simulink model "VSD_Model"  (R2022a)
settings: Solver=VariableStepAuto  StartTime=0.0  StopTime=60
values from neighbouring files (symbols this model uses):
  Bm = 7.33*10^-8/(2*pi)    (= 1.16660573286e-08)    [VSD_Motors_initialization.m]
  fit_Cp_tail = @(u)feval(f_Cp_tail,u)    [VSD_Propellerfitting_tail.m]
  fit_Ct_tail = @(u)feval(f_Ct_tail,u)    [VSD_Propellerfitting_tail.m]
  fit_Pe_tail = @(u)feval(f_Pe_tail,u)    [VSD_Propellerfitting_tail.m]
  fit_Tl_tail = @(u)feval(f_Tl_tail,u)    [VSD_Propellerfitting_tail.m]
  Jm = 1.72 *10^-6    (= 1.72e-06)    [VSD_Motors_initialization.m]
  Ke = Km    (= 0.00118)    [VSD_Motors_initialization.m]
  Km = 1.18*10^-3    (= 0.00118)    [VSD_Motors_initialization.m]
  La = 0.274*10^-3    (= 0.000274)    [VSD_Motors_initialization.m]
  Q = 1e-6    (= 1e-06)    [VSD_initialization.m]
  R = 0.486    [VSD_Motors_initialization.m]    (also in VSD_initialization.m = 0.001)
  Ts = 1e-4    (= 0.0001)    [VSD_initialization.m]    (also in myStateTransitionFcn.m = 0.01)
  x0 = [0;0;0;0;0;0;0;0;0;0;0;0]    [VSD_SystemCheck.m]    (also in VSD_initialization.m = [0,0,0,0,0,0,0,0,0,0,0,0])
undefined symbols (not defined in the file or in its folder): Continuous, Time
libraries: slpidlib x7, simulink x7, sharedTrackingLibrary x3, ctrlSharedLib x1
(part 1 of 2)
settings Model: Creator=luca9  LastModifiedBy=luca9
settings SolverCC: AlgebraicLoopSolver=TrustRegion
settings DebuggingCC: UnconnectedInputMsg=warning  UnconnectedOutputMsg=warning  UnconnectedLineMsg=warning
settings RTWCC: DLArmComputeVersion=19.05

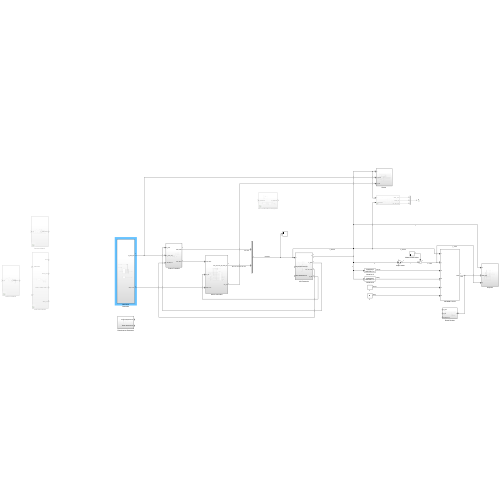
[thumbnail: Simulink's stored preview of the top-level diagram]
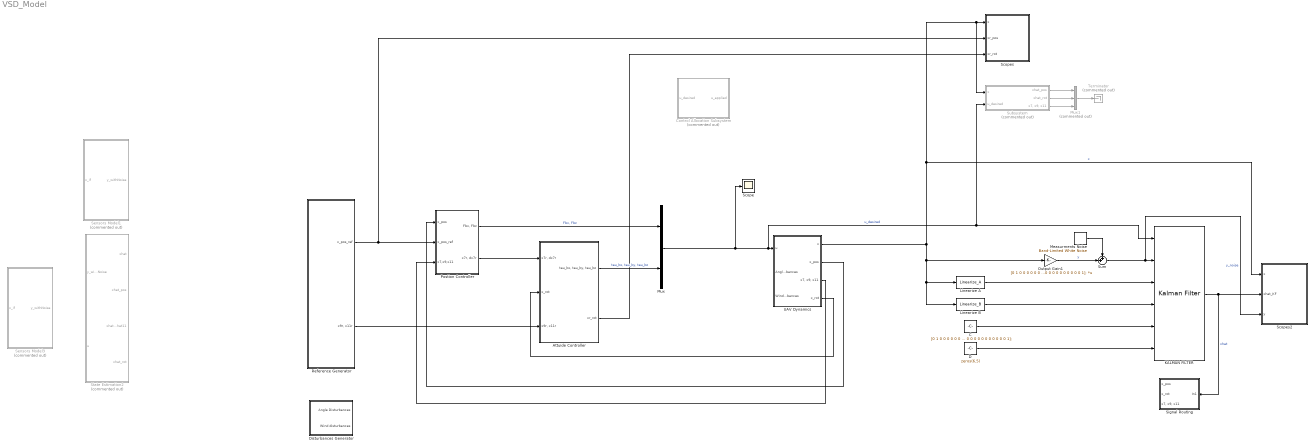
== system VSD_Model ==
  Attuide Controller : Subsystem
  C : Constant  Value=|  VectorParams1D=off
      | [0 1 0 0 0 0 0 0 0 0 0 0;
      |      0 0 0 1 0 0 0 0 0 0 0 0;
      |      0 0 0 0 0 1 0 0 0 0 0 0;
      |      0 0 0 0 0 0 0 1 0 0 0 0;
      |      0 0 0 0 0 0 0 0 0 1 0 0;
      |      0 0 0 0 0 0 0 0 0 0 0 1];
  Control Allocation Subsystem : Subsystem  Commented=on
  D : Constant  Value=zeros(6,5)  VectorParams1D=off
  Disturbances Generator : Subsystem
  KALMAN FILTER : ctrlSharedLib/Kalman Filter  TimeDomain=Continuous-Time  UseCurrentEstimator=on  ModelSource=Input port  ModelSourceVariable=ss(0.95,1,1,0,1)  A=0.95  B=1  C=1  D=0  NumberOfStates=12  NumberOfInputs=5  NumberOfOutputs=6  InitialEstimateSource=Dialog  X0=x0  P0=10^-2*eye(12)  UseK=off  UseGH=off  NumberOfProcessNoiseInputs=1  G=1  TimeInvariantG=on  H=0  TimeInvariantH=on  Q=Q*eye(12)  TimeInvariantQ=on  R=R*eye(6)  TimeInvariantR=on  N=0  TimeInvariantN=on  AddInputPort=on  AddEnablePort=off  OutputEstimatedY=off  OutputP=off  Ts=-1
  Linearize A : MATLABFcn  MATLABFcn=Linearize_A  OutputDimensions=[12,12]  Output1D=off
  Linearize B : MATLABFcn  MATLABFcn=Linearize_B  OutputDimensions=[12,5]  Output1D=off
  "Measurments Noise " : simulink/Sources/Band-Limited White Noise  Cov=R*Ts  Ts=Ts  seed=[23341]
  Mux : Mux  Inputs=2
  Mux1 : Mux  Commented=on  Inputs=3
  Output Gain1 : Gain  Gain=|  Multiplication=Matrix(K*u)
      | [0 1 0 0 0 0 0 0 0 0 0 0;
      |      0 0 0 1 0 0 0 0 0 0 0 0;
      |      0 0 0 0 0 1 0 0 0 0 0 0;
      |      0 0 0 0 0 0 0 1 0 0 0 0;
      |      0 0 0 0 0 0 0 0 0 1 0 0;
      |      0 0 0 0 0 0 0 0 0 0 0 1];
  Postion Controller : Subsystem
  Reference Generator : Subsystem
  Scope : Scope
  Scopes : Subsystem
  Scopes2 : Subsystem
  Sensors Model1 : Subsystem  Commented=on
  Sensors Model3 : Subsystem  Commented=on
  Signal Routing : Subsystem
  State Estimation2 : Subsystem  Commented=on
  Subsystem : Subsystem  Commented=on
  Sum : Sum  Inputs=++|
  Terminator : Terminator  Commented=on
  UAV Dynamics : Subsystem
  wires:
  Postion Controller/2("x7r, dx7r") -> Attuide Controller/1("x7r, dx7r")
  Mux/1 -> Scope/1, Subsystem/2(u_desired), KALMAN FILTER/1, UAV Dynamics/1(u)  "u_desired"
  Attuide Controller/1("tau_bx, tau_by, tau_bz") -> Mux/2  "tau_bx, tau_by, tau_bz"
  Postion Controller/1("Fbx, Fbz") -> Mux/1  "Fbx, Fbz"
  Reference Generator/1(x_pos_ref) -> Scopes/2(xr_pos), Postion Controller/2(x_pos_ref)
  Reference Generator/2("x9r, x11r") -> Attuide Controller/3("x9r, x11r")
  UAV Dynamics/1(x) -> Subsystem/1(x), Scopes/1(x), Scopes2/1(x), Output Gain1/1, Linearize B/1, Linearize A/1  "x"
  Attuide Controller/2(xr_rot) -> Scopes/3(xr_rot)
  Linearize A/1 -> KALMAN FILTER/3
  Linearize B/1 -> KALMAN FILTER/4
  D/1 -> KALMAN FILTER/6
  KALMAN FILTER/1 -> Scopes2/2(xhat_KF), Signal Routing/1(In1)  "xhat"
  Output Gain1/1 -> Sum/2  "y"
  Sum/1 -> Scopes2/3(y), KALMAN FILTER/2  "y_noise"
  "Measurments Noise "/1 -> Sum/1
  Subsystem/2(xhat_rot) -> Mux1/2
  Subsystem/1(xhat_pos) -> Mux1/1
  Subsystem/3("x7, x9, x11") -> Mux1/3
  Mux1/1 -> Terminator/1
  C/1 -> KALMAN FILTER/5
  UAV Dynamics/2(x_pos) -> Postion Controller/1(x_pos)
  UAV Dynamics/4(x_rot) -> Attuide Controller/2(x_rot)
  UAV Dynamics/3("x7, x9, x11") -> Postion Controller/3(" x7,x9,x11")

== system VSD_Model/Attuide Controller ==
  "x7r, dx7r" : Inport
  x_rot : Inport  Port=2
  "x9r, x11r" : Inport  Port=3
  Attitude Controller : MATLAB Function  TreatAsAtomicUnit=on
  Constant : Constant  Value=0
  Constant1 : Constant  Value=0
  Demux : Demux  Outputs=2
  Demux1 : Demux  Outputs=2
  Mux : Mux  Inputs=3
  Mux1 : Mux  Inputs=6
  Scope : Scope
  To Workspace : ToWorkspace  VariableName=s  SampleTime=-1
  "tau_bx, tau_by, tau_bz" : Outport
  xr_rot : Outport  Port=2
  wires:
  x_rot/1 -> Attitude Controller/1(x_rot)
  "x7r, dx7r"/1 -> Demux/1
  Demux/1 -> Attitude Controller/2(x7r), Mux1/1  "x7r"
  Demux/2 -> Attitude Controller/3(dx7r), Mux1/2  "dx7r"
  Demux1/1 -> Attitude Controller/4(x9r), Mux1/3  "x9r"
  "x9r, x11r"/1 -> Demux1/1
  Demux1/2 -> Mux1/5, Attitude Controller/6(x11r)
  Constant/1 -> Attitude Controller/5(dx9r), Mux1/4  "dx9r"
  Constant1/1 -> Attitude Controller/7(dx11r), Mux1/6
  Mux/1 -> "tau_bx, tau_by, tau_bz"/1
  Attitude Controller/2(u5) -> Mux/2
  Attitude Controller/1(u4) -> Mux/1
  Attitude Controller/3(u6) -> Mux/3
  Mux1/1 -> xr_rot/1
  Attitude Controller/4(s) -> To Workspace/1, Scope/1

== system VSD_Model/Control Allocation Subsystem ==
  u_desired : Inport
  Control allocation : Subsystem  Commented=on
  DC Motors : Subsystem  Commented=on
  Mux3 : Mux  Commented=on  Inputs=2
  Mux4 : Mux  Commented=on
  Scope1 : Scope  Commented=on  NumInputPorts=2
  Step{1..6} (6 alike) : Step  Commented=on  Time=0  After=0  SampleTime=0
  u_applied : Outport
  wires:
  DC Motors/1(y) -> Scope1/2, u_applied/1  "u_applied"
  Control allocation/7(alpha_r) -> DC Motors/7(alpha_r)
  Control allocation/2(W2) -> DC Motors/2(W2)
  Control allocation/6(alpha_l) -> DC Motors/6(alpha_l)
  Step4/1 -> Mux4/2
  Step6/1 -> Mux4/4
  u_desired/1 -> Control allocation/1(u), Scope1/1
  Control allocation/4(W4) -> DC Motors/4(W4)
  Control allocation/5(W5) -> DC Motors/5(W5)
  Control allocation/3(W3) -> DC Motors/3(W3)
  Step5/1 -> Mux4/3
  Control allocation/1(W1) -> DC Motors/1(w1)  "w1"
  Mux3/1 -> DC Motors/9(Tload_servo)
  Mux4/1 -> DC Motors/8(Tload_motor2)
  Step3/1 -> Mux3/2
  Step1/1 -> Mux4/1
  Step2/1 -> Mux3/1

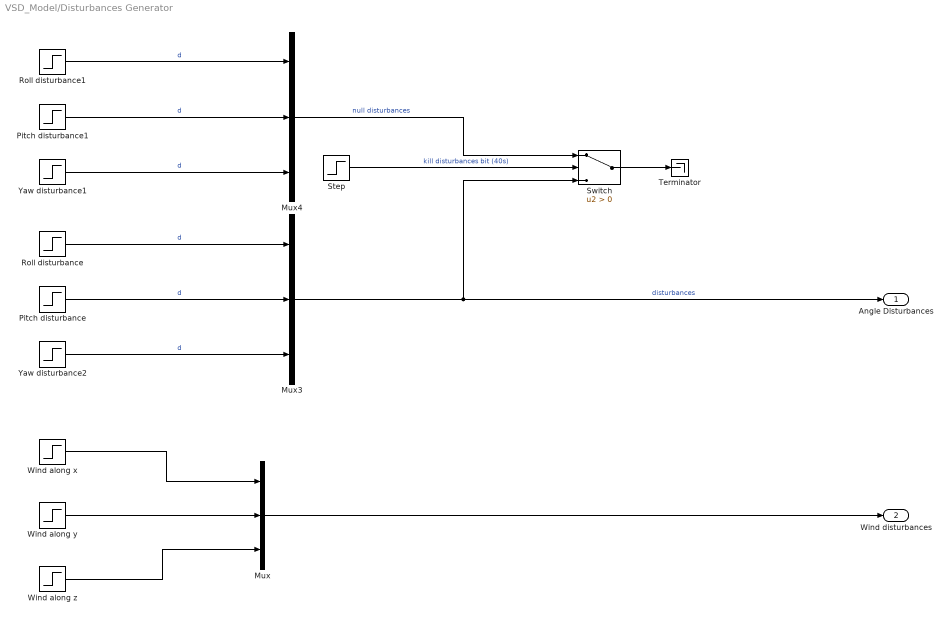
== system VSD_Model/Disturbances Generator ==
  Mux : Mux  Inputs=3
  Mux3 : Mux  Inputs=3
  Mux4 : Mux  Inputs=3
  Pitch disturbance : Step  Time=20  After=0.5  SampleTime=0
  Pitch disturbance1 : Step  Time=0  After=0  SampleTime=0
  Roll disturbance : Step  Time=10  After=0.5  SampleTime=0
  Roll disturbance1 : Step  Time=0  After=0  SampleTime=0
  Step : Step  Time=90  SampleTime=0
  Switch : Switch  Criteria=u2 > Threshold  SaturateOnIntegerOverflow=off  InputSameDT=off
  Terminator : Terminator
  Wind along x : Step  Time=0  SampleTime=0
  Wind along y : Step  Time=0  SampleTime=0
  Wind along z : Step  Time=0  After=0  SampleTime=0
  Yaw disturbance1 : Step  Time=0  After=0  SampleTime=0
  Yaw disturbance2 : Step  Time=30  After=0.25  SampleTime=0
  Angle Disturbances : Outport
  Wind disturbances : Outport  Port=2
  wires:
  Pitch disturbance/1 -> Mux3/2  "d"
  Yaw disturbance1/1 -> Mux4/3  "d"
  Yaw disturbance2/1 -> Mux3/3  "d"
  Pitch disturbance1/1 -> Mux4/2  "d"
  Roll disturbance/1 -> Mux3/1  "d"
  Mux3/1 -> Switch/3, Angle Disturbances/1  "disturbances"
  Step/1 -> Switch/2  "kill disturbances bit (40s)"
  Roll disturbance1/1 -> Mux4/1  "d"
  Mux4/1 -> Switch/1  "null disturbances"
  Switch/1 -> Terminator/1
  Wind along y/1 -> Mux/2
  Wind along x/1 -> Mux/1
  Wind along z/1 -> Mux/3
  Mux/1 -> Wind disturbances/1

== system VSD_Model/Postion Controller ==
  x_pos : Inport
  x_pos_ref : Inport  Port=2
  " x7,x9,x11" : Inport  Port=3
  Decoupler : MATLAB Function  TreatAsAtomicUnit=on
  Demux : Demux  Outputs=3
  Derivative : Derivative
  Mass : Gain  Gain=1.331
  Mux1 : Mux  Inputs=3
  Mux2 : Mux  Inputs=2
  Mux3 : Mux  Inputs=2
  To Workspace : ToWorkspace  VariableName=x7r  SampleTime=-1
  Virtual  Controller : MATLAB Function  TreatAsAtomicUnit=on
  "Fbx, Fbz" : Outport
  "x7r, dx7r" : Outport  Port=2
  wires:
  x_pos_ref/1 -> Virtual  Controller/1(xref)
  x_pos/1 -> Virtual  Controller/2(x_pos)
  Virtual  Controller/1(u1d) -> Mux1/1
  Virtual  Controller/2(u2d) -> Mux1/2
  Virtual  Controller/3(u3d) -> Mux1/3
  Mux1/1 -> Decoupler/1(ud)
  Decoupler/1(x7r) -> To Workspace/1, Derivative/1, Mux3/1  "req roll angle"
  Decoupler/2(ux) -> Mux2/1
  Decoupler/3(uz) -> Mux2/2
  " x7,x9,x11"/1 -> Demux/1
  Demux/1 -> Decoupler/2(x7)
  Demux/2 -> Decoupler/3(x9)
  Demux/3 -> Decoupler/4(x11)
  Derivative/1 -> Mux3/2
  Mux3/1 -> "x7r, dx7r"/1
  Mux2/1 -> Mass/1  "ux, uz"
  Mass/1 -> "Fbx, Fbz"/1  "Fbx, Fbz"

== system VSD_Model/Reference Generator ==
  Clock : Clock
      settings: Decimation=3
  Mux1 : Mux  Inputs=9
  Mux2 : Mux  Inputs=3
  Pitch Yaw Reference Generator : Subsystem
  Position References (HELIX / RAMP) : MATLAB Function  TreatAsAtomicUnit=on
  To Workspace : ToWorkspace  VariableName=ref  SampleTime=-1
  To Workspace1 : ToWorkspace  VariableName=t  SampleTime=-1
  x_pos_ref : Outport
  "x9r, x11r" : Outport  Port=2
  wires:
  Position References (HELIX / RAMP)/4(y_des) -> Mux1/4, Mux2/2
  Position References (HELIX / RAMP)/5(dy_des) -> Mux1/5
  Position References (HELIX / RAMP)/8(dz_des) -> Mux1/8
  Position References (HELIX / RAMP)/7(z_des) -> Mux1/7, Mux2/3
  Position References (HELIX / RAMP)/9(ddz_des) -> Mux1/9
  Position References (HELIX / RAMP)/1(x_des) -> Mux1/1, Mux2/1
  Position References (HELIX / RAMP)/6(ddy_des) -> Mux1/6
  Position References (HELIX / RAMP)/2(dx_des) -> Mux1/2
  Mux2/1 -> To Workspace/1
  Position References (HELIX / RAMP)/3(ddx_des) -> Mux1/3
  Clock/1 -> Position References (HELIX / RAMP)/1(t), To Workspace1/1
  Pitch Yaw Reference Generator/1("x9r, x11r") -> "x9r, x11r"/1  "x9r, x11r"
  Mux1/1 -> x_pos_ref/1

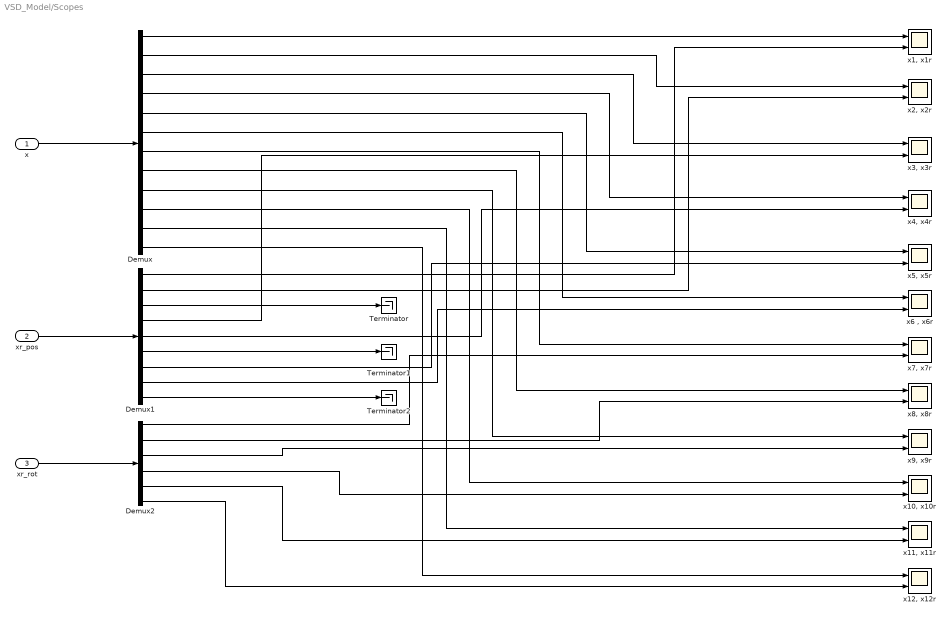
== system VSD_Model/Scopes ==
  x : Inport
  xr_pos : Inport  Port=2
  xr_rot : Inport  Port=3
  Demux : Demux  Outputs=12
  Demux1 : Demux  Outputs=9
  Demux2 : Demux  Outputs=6
  Terminator : Terminator
  Terminator1 : Terminator
  Terminator2 : Terminator
  "x1, x1r" : Scope  NumInputPorts=2
  "x10, x10r" : Scope  NumInputPorts=2
  "x11, x11r" : Scope  NumInputPorts=2
  "x12, x12r" : Scope  NumInputPorts=2
  "x2, x2r" : Scope  NumInputPorts=2
  "x3, x3r" : Scope  NumInputPorts=2
  "x4, x4r" : Scope  NumInputPorts=2
  "x5, x5r" : Scope  NumInputPorts=2
  "x6 , x6r" : Scope  NumInputPorts=2
  "x7, x7r" : Scope  NumInputPorts=2
  "x8, x8r" : Scope  NumInputPorts=2
  "x9, x9r" : Scope  NumInputPorts=2
  wires:
  xr_pos/1 -> Demux1/1
  x/1 -> Demux/1
  Demux/1 -> "x1, x1r"/1
  Demux1/9 -> Terminator2/1
  Demux1/6 -> Terminator1/1
  Demux1/3 -> Terminator/1
  Demux1/1 -> "x1, x1r"/2
  xr_rot/1 -> Demux2/1
  Demux/2 -> "x2, x2r"/1
  Demux/3 -> "x3, x3r"/1
  Demux/4 -> "x4, x4r"/1
  Demux/5 -> "x5, x5r"/1
  Demux/6 -> "x6 , x6r"/1
  Demux/7 -> "x7, x7r"/1
  Demux/8 -> "x8, x8r"/1
  Demux/9 -> "x9, x9r"/1
  Demux/10 -> "x10, x10r"/1
  Demux/11 -> "x11, x11r"/1
  Demux/12 -> "x12, x12r"/1
  Demux1/2 -> "x2, x2r"/2
  Demux1/7 -> "x5, x5r"/2
  Demux1/8 -> "x6 , x6r"/2
  Demux2/1 -> "x7, x7r"/2
  Demux2/2 -> "x8, x8r"/2
  Demux2/3 -> "x9, x9r"/2
  Demux2/4 -> "x10, x10r"/2
  Demux2/5 -> "x11, x11r"/2
  Demux2/6 -> "x12, x12r"/2
  Demux1/4 -> "x3, x3r"/2
  Demux1/5 -> "x4, x4r"/2

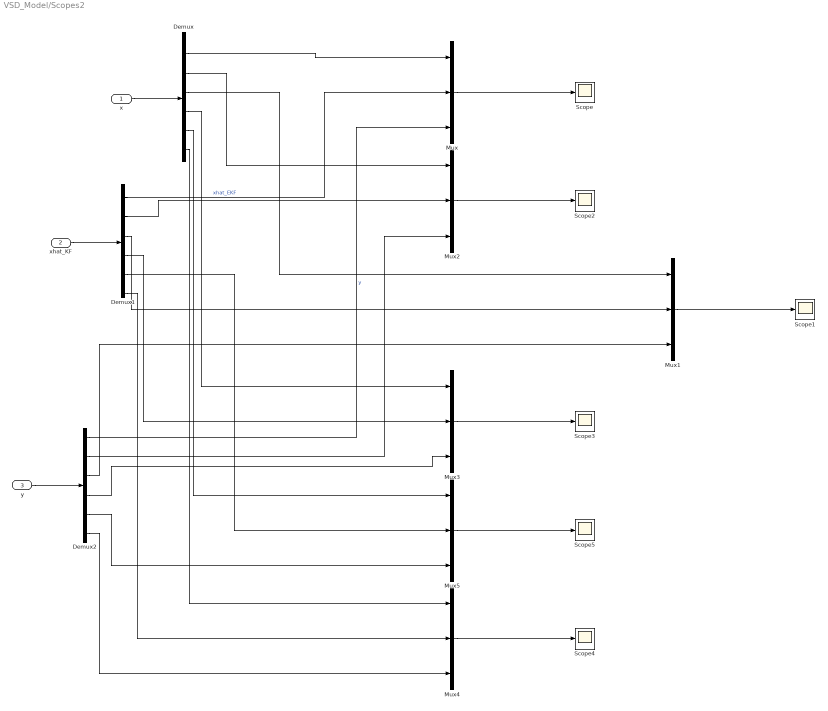
== system VSD_Model/Scopes2 ==
  x : Inport
  xhat_KF : Inport  Port=2
  y : Inport  Port=3
  Demux : Demux  Outputs=12
  Demux1 : Demux  Outputs=12
  Demux2 : Demux  Outputs=6
  Mux{,1..5} (6 alike) : Mux  Inputs=3
  Scope{,1..5} (6 alike) : Scope
  wires:
  x/1 -> Demux/1
  xhat_KF/1 -> Demux1/1
  Demux/2 -> Mux/1
  Demux1/2 -> Mux/2  "xhat_EKF"
  Mux/1 -> Scope/1
  y/1 -> Demux2/1
  Demux2/1 -> Mux/3  "y"
  Mux1/1 -> Scope1/1
  Demux/6 -> Mux1/1
  Demux1/6 -> Mux1/2
  Demux2/3 -> Mux1/3
  Mux2/1 -> Scope2/1
  Demux/4 -> Mux2/1
  Demux1/4 -> Mux2/2
  Demux2/2 -> Mux2/3
  Mux5/1 -> Scope5/1
  Mux4/1 -> Scope4/1
  Mux3/1 -> Scope3/1
  Demux/8 -> Mux3/1
  Demux/10 -> Mux5/1
  Demux/12 -> Mux4/1
  Demux1/8 -> Mux3/2
  Demux1/10 -> Mux5/2
  Demux1/12 -> Mux4/2
  Demux2/4 -> Mux3/3
  Demux2/5 -> Mux5/3
  Demux2/6 -> Mux4/3

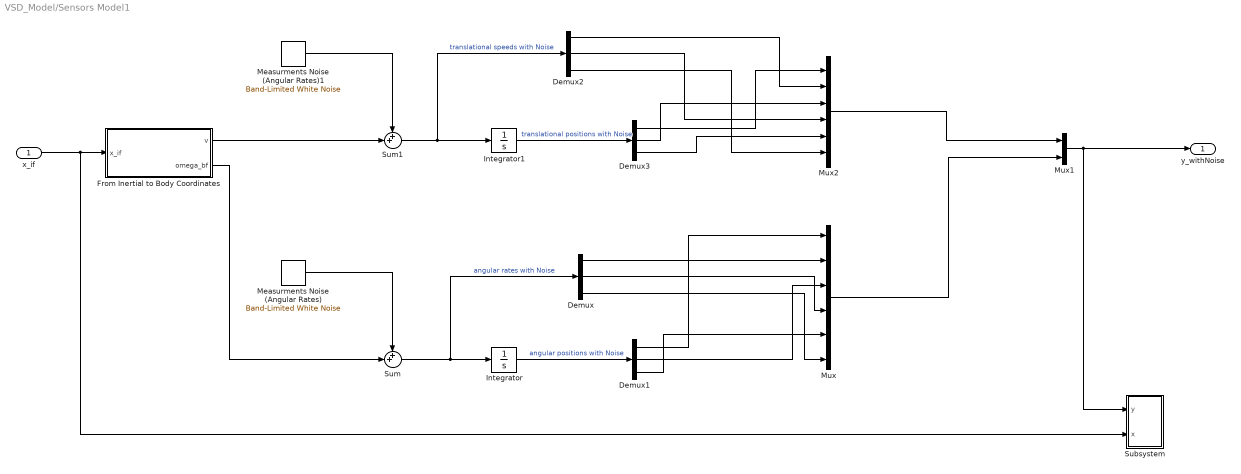
== system VSD_Model/Sensors Model1 ==
  x_if : Inport
  Demux{,1..3} (4 alike) : Demux  Outputs=3
  From Inertial to Body Coordinates : MATLAB Function  TreatAsAtomicUnit=on
  Integrator : Integrator
  Integrator1 : Integrator
  Measurments Noise (Angular Rates) : simulink/Sources/Band-Limited White Noise  Cov=R*Ts  Ts=Ts  seed=[23341]
  Measurments Noise (Angular Rates)1 : simulink/Sources/Band-Limited White Noise  Cov=R*Ts  Ts=Ts  seed=[23341]
  Mux : Mux  Inputs=6
  Mux1 : Mux  Inputs=2
  Mux2 : Mux  Inputs=6
  Subsystem : Subsystem
  Sum : Sum  Inputs=++|
  Sum1 : Sum  Inputs=++|
  y_withNoise : Outport
  wires:
  x_if/1 -> From Inertial to Body Coordinates/1(x_if), Subsystem/2(x)
  From Inertial to Body Coordinates/2(omega_bf) -> Sum/2
  Sum/1 -> Integrator/1, Demux/1  "angular rates with Noise"
  Demux/1 -> Mux/2
  Demux/2 -> Mux/4
  Demux/3 -> Mux/6
  Integrator/1 -> Demux1/1  "angular positions with Noise"
  Demux1/1 -> Mux/1
  Demux1/2 -> Mux/3
  Demux1/3 -> Mux/5
  Mux/1 -> Mux1/2
  From Inertial to Body Coordinates/1(v) -> Sum1/2
  Sum1/1 -> Demux2/1, Integrator1/1  "translational speeds with Noise"
  Integrator1/1 -> Demux3/1  "translational positions with Noise"
  Demux2/3 -> Mux2/6
  Demux2/2 -> Mux2/4
  Demux2/1 -> Mux2/2
  Demux3/1 -> Mux2/1
  Demux3/2 -> Mux2/3
  Demux3/3 -> Mux2/5
  Mux2/1 -> Mux1/1
  Mux1/1 -> Subsystem/1(y), y_withNoise/1
  Measurments Noise (Angular Rates)1/1 -> Sum1/1
  Measurments Noise (Angular Rates)/1 -> Sum/1

== system VSD_Model/Sensors Model3 ==
  x_if : Inport
  Body 2 Inertial : MATLAB Function  TreatAsAtomicUnit=on
  Demux : Demux  Outputs=12
  Demux1 : Demux  Outputs=3
  Demux2 : Demux  Outputs=3
  From Body to Inertial Coordinates : MATLAB Function  TreatAsAtomicUnit=on
  From Inertial to Body Coordinates : MATLAB Function  TreatAsAtomicUnit=on
  Measurments Noise (Angular Rates) : simulink/Sources/Band-Limited White Noise  Cov=R*Ts  Ts=Ts  seed=[23341]
  Measurments Noise (Angular Rates)1 : simulink/Sources/Band-Limited White Noise  Cov=R*Ts  Ts=Ts  seed=[23341]
  Mux : Mux  Inputs=12
  Mux1 : Mux  Inputs=6
  Sum : Sum  Inputs=++|
  Sum1 : Sum  Inputs=++|
  y_withNoise : Outport
  wires:
  x_if/1 -> From Inertial to Body Coordinates/1(x_if), From Body to Inertial Coordinates/2(x_if), Body 2 Inertial/2(x_if), Demux/1
  From Inertial to Body Coordinates/2(omega_bf) -> Sum/2
  From Inertial to Body Coordinates/1(v_bf) -> Sum1/2
  Measurments Noise (Angular Rates)1/1 -> Sum1/1
  Measurments Noise (Angular Rates)/1 -> Sum/1
  Sum1/1 -> From Body to Inertial Coordinates/1(u)  "translational speeds with Noise"
  Sum/1 -> Body 2 Inertial/1(u)  "angular rates with Noise"
  From Body to Inertial Coordinates/1(y) -> Demux1/1
  Body 2 Inertial/1(y) -> Demux2/1
  Demux2/3 -> Mux1/6, Mux/12
  Demux2/2 -> Mux/10, Mux1/5
  Demux2/1 -> Mux/8, Mux1/4
  Demux/11 -> Mux/11
  Demux/9 -> Mux/9
  Demux/7 -> Mux/7
  Demux/1 -> Mux/1
  Demux/3 -> Mux/3
  Demux/5 -> Mux/5
  Demux1/1 -> Mux1/1, Mux/2
  Demux1/2 -> Mux/4, Mux1/2
  Demux1/3 -> Mux/6, Mux1/3
  Mux1/1 -> y_withNoise/1

== system VSD_Model/Signal Routing ==
  In1 : Inport
  Demux : Demux  Outputs=2
  Demux1 : Demux  Outputs=6
  Mux : Mux  Inputs=3
  x_pos : Outport
  x_rot : Outport  Port=2
  "x7, x9, x11" : Outport  Port=3
  wires:
  In1/1 -> Demux/1
  Demux/1 -> x_pos/1
  Demux/2 -> Demux1/1, x_rot/1
  Mux/1 -> "x7, x9, x11"/1
  Demux1/1 -> Mux/1
  Demux1/3 -> Mux/2
  Demux1/5 -> Mux/3

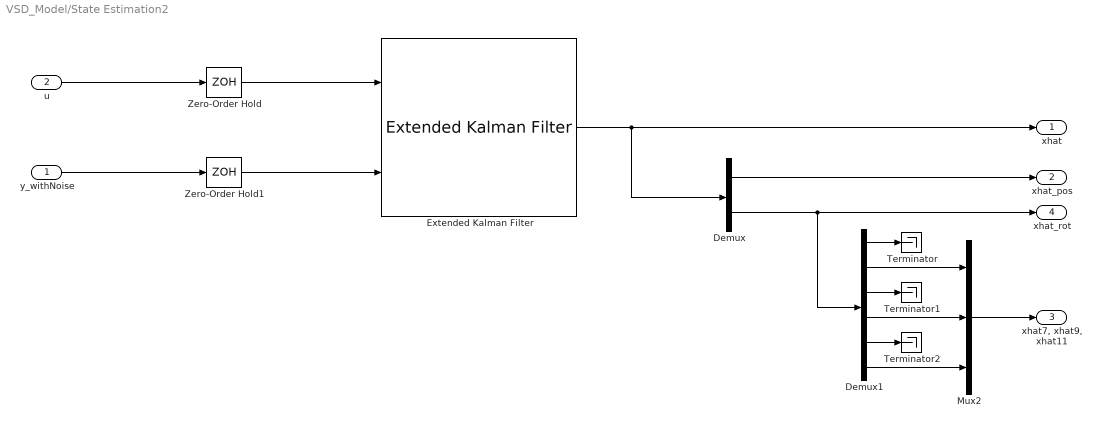
== system VSD_Model/State Estimation2 ==
  y_withNoise : Inport
  u : Inport  Port=2
  Demux : Demux  Outputs=2
  Demux1 : Demux  Outputs=6
  Extended Kalman Filter : sharedTrackingLibrary/Extended Kalman Filter  StateTransitionFcn=myStateTransitionFcn  HasStateTransitionJacobianFcn=off  HasAdditiveProcessNoise=Additive  ProcessNoise=Q*eye(12)  HasTimeVaryingProcessNoise=off  HasStateTransitionFcnExtraArgument=1  InitialState=x0  InitialStateCovariance=1e-3  MeasurementFcn1=myMeasurementFcn  HasMeasurementJacobianFcn1=off  HasMeasurementEnablePort1=off  HasAdditiveMeasurementNoise1=Additive  MeasurementNoise1=R*eye(12)  HasTimeVaryingMeasurementNoise1=off  HasMeasurementFcnExtraArgument1=0  HasMeasurementWrapping1=off  MeasurementFcn2=myMeasurementFcn  HasMeasurementJacobianFcn2=off  HasMeasurementEnablePort2=off  HasAdditiveMeasurementNoise2=Additive  MeasurementNoise2=1  HasTimeVaryingMeasurementNoise2=off  HasMeasurementFcnExtraArgument2=0  HasMeasurementWrapping2=off  MeasurementFcn3=myMeasurementFcn  HasMeasurementJacobianFcn3=off  HasMeasurementEnablePort3=off  HasAdditiveMeasurementNoise3=Additive  MeasurementNoise3=1  HasTimeVaryingMeasurementNoise3=off  HasMeasurementFcnExtraArgument3=0  HasMeasurementWrapping3=off  MeasurementFcn4=myMeasurementFcn  HasMeasurementJacobianFcn4=off  HasMeasurementEnablePort4=off  HasAdditiveMeasurementNoise4=Additive  MeasurementNoise4=1  HasTimeVaryingMeasurementNoise4=off  HasMeasurementFcnExtraArgument4=0  HasMeasurementWrapping4=off  MeasurementFcn5=myMeasurementFcn  HasMeasurementJacobianFcn5=off  HasMeasurementEnablePort5=off  HasAdditiveMeasurementNoise5=Additive  MeasurementNoise5=1  HasTimeVaryingMeasurementNoise5=off  HasMeasurementFcnExtraArgument5=0  HasMeasurementWrapping5=off  EnableMultirate=off  StateTransitionFcnSampleTime=1  MeasurementFcn1SampleTime=1  MeasurementFcn2SampleTime=1  MeasurementFcn3SampleTime=1  MeasurementFcn4SampleTime=1  MeasurementFcn5SampleTime=1  UseCurrentEstimator=on  OutputStateCovariance=off  DataType=double  SampleTime=Ts  NumberOfMeasurements=1
      settings: SourceProductBaseCode=TF,AE,PW,CT,DR,ID,LP,NV,AR,RO,RR,UV,VE
  Mux2 : Mux  Inputs=3
  Terminator : Terminator
  Terminator1 : Terminator
  Terminator2 : Terminator
  Zero-Order Hold : ZeroOrderHold  SampleTime=Ts
  Zero-Order Hold1 : ZeroOrderHold  SampleTime=Ts
  xhat : Outport
  xhat_pos : Outport  Port=2
  "xhat7, xhat9, xhat11" : Outport  Port=3
  xhat_rot : Outport  Port=4
  wires:
  u/1 -> Zero-Order Hold/1
  Zero-Order Hold/1 -> Extended Kalman Filter/1
  y_withNoise/1 -> Zero-Order Hold1/1
  Zero-Order Hold1/1 -> Extended Kalman Filter/2
  Extended Kalman Filter/1 -> xhat/1, Demux/1
  Demux/1 -> xhat_pos/1
  Demux/2 -> xhat_rot/1, Demux1/1
  Demux1/1 -> Terminator/1
  Demux1/3 -> Terminator1/1
  Demux1/5 -> Terminator2/1
  Demux1/2 -> Mux2/1
  Demux1/4 -> Mux2/2
  Demux1/6 -> Mux2/3
  Mux2/1 -> "xhat7, xhat9, xhat11"/1

== system VSD_Model/Subsystem ==
  x : Inport
  u_desired : Inport  Port=2
  Scopes1 : Subsystem  Commented=on
  Sensors Model2 : Subsystem  Commented=on
  State Estimation1 : Subsystem  Commented=on
  xhat_pos : Outport
  xhat_rot : Outport  Port=2
  "x7, x9, x11" : Outport  Port=3
  wires:
  u_desired/1 -> State Estimation1/2(u)
  State Estimation1/1(xhat_EKF) -> Scopes1/3(xhat_EKF)
  State Estimation1/2(xhat_UKF) -> Scopes1/4(xhat_UKF)
  Sensors Model2/1(y_withNoise) -> Scopes1/2(y), State Estimation1/1(y_withNoise)  "y"
  x/1 -> Sensors Model2/1(x_if), Scopes1/1(x)
  State Estimation1/5("x7, x9, x11") -> "x7, x9, x11"/1
  State Estimation1/3(xhat_pos) -> xhat_pos/1
  State Estimation1/4(xhat_rot) -> xhat_rot/1

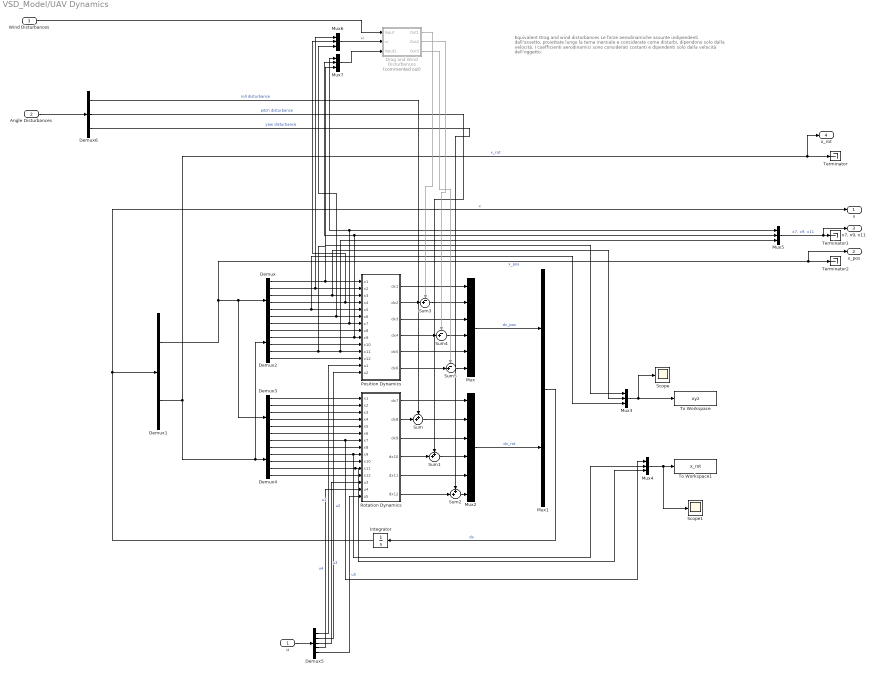
== system VSD_Model/UAV Dynamics ==
  note: Equivalent Drag and wind disturbances
      | Le forze aerodinamiche assunte indipendenti dall'assetto, proiettate lungo la terna inerziale e considerate come disturbi, dipendono solo dalla velocità.
      | I coefficienti aerodinamici sono considerati costanti e dipendenti solo dalla velocità dell'oggetto.
  u : Inport
  Angle Disturbances : Inport  Port=2
  Wind Disturbances : Inport  Port=3
  Demux{,2..4} (4 alike) : Demux  Outputs=6
  Demux1 : Demux  Outputs=2
  Demux5 : Demux  Outputs=5
  Demux6 : Demux  Outputs=3
  Drag and Wind Disturbances : Subsystem  Commented=on
  Integrator : Integrator  InitialCondition=[0;0;0;0;0;0;0;0;0;0;0;0]  UpperSaturationLimit=[inf; 10; inf; 10; inf; 10; 0.1; 0.5; 1; 2; 0.01; 0.1]  LowerSaturationLimit=[-inf; -10; -inf; -10; -inf; -10; -0.1; -0.5; -1; -2; -0.01; -0.1]
  Mux : Mux  Inputs=6
  Mux1 : Mux  Inputs=2
  Mux2 : Mux  Inputs=6
  Mux{3..7} (5 alike) : Mux  Inputs=3
  Position Dynamics : MATLAB Function  TreatAsAtomicUnit=on
  Rotation Dynamics : MATLAB Function  TreatAsAtomicUnit=on
  Scope : Scope
  Scope1 : Scope
  Sum : Sum  Inputs=++|
  Sum1 : Sum  Inputs=++|
  Sum2 : Sum  Inputs=++|
  Sum3 : Sum  Inputs=-+|
  Sum4 : Sum  Inputs=-+|
  Sum5 : Sum  Inputs=-+|
  Terminator : Terminator
  Terminator1 : Terminator
  Terminator2 : Terminator
  To Workspace : ToWorkspace  VariableName=xyz  SampleTime=-1
  To Workspace1 : ToWorkspace  VariableName=x_rot  SampleTime=-1
  x : Outport
  x_pos : Outport  Port=2
  "x7, x9, x11" : Outport  Port=3
  x_rot : Outport  Port=4
  wires:
  Position Dynamics/5(dx5) -> Mux/5
  Demux3/4 -> Rotation Dynamics/4(x4)
  Demux/4 -> Position Dynamics/4(x4), Mux6/2
  Demux3/2 -> Rotation Dynamics/2(x2)
  Demux1/2 -> Demux2/1, Demux4/1, Terminator/1, x_rot/1  "x_rot"
  Demux/5 -> Mux3/3, Position Dynamics/5(x5)
  Demux2/6 -> Position Dynamics/12(x12)
  Rotation Dynamics/1(dx7) -> Mux2/1
  Demux3/1 -> Rotation Dynamics/1(x1)
  Demux4/1 -> Mux4/1, Rotation Dynamics/7(x7)
  Demux5/1 -> Position Dynamics/13(u1)  "u1"
  Demux4/4 -> Rotation Dynamics/10(x10)
  Demux2/5 -> Position Dynamics/11(x11), Mux5/3, Mux7/3
  Demux2/1 -> Mux5/1, Mux7/1, Position Dynamics/7(x7)
  Demux4/5 -> Mux4/3, Rotation Dynamics/11(x11)
  Demux/2 -> Position Dynamics/2(x2), Mux6/1
  Mux2/1 -> Mux1/2  "dx_rot"
  Demux/1 -> Mux3/1, Position Dynamics/1(x1)
  Demux4/3 -> Mux4/2, Rotation Dynamics/9(x9)
  Demux3/6 -> Rotation Dynamics/6(x6)
  Demux/6 -> Position Dynamics/6(x6), Mux6/3
  Demux5/2 -> Position Dynamics/14(u2)  "u2"
  Demux2/4 -> Position Dynamics/10(x10)
  Demux5/4 -> Rotation Dynamics/14(u4)  "u4"
  Demux5/5 -> Rotation Dynamics/15(u5)  "u5"
  Demux/3 -> Mux3/2, Position Dynamics/3(x3)
  u/1 -> Demux5/1
  Mux/1 -> Mux1/1  "dx_pos"
  Demux2/3 -> Mux5/2, Mux7/2, Position Dynamics/9(x9)
  Demux2/2 -> Position Dynamics/8(x8)
  Integrator/1 -> x/1, Demux1/1  "x"
  Demux1/1 -> x_pos/1, Terminator2/1, Demux/1, Demux3/1  "x_pos"
  Demux5/3 -> Rotation Dynamics/13(u3)  "u3"
  Position Dynamics/3(dx3) -> Mux/3
  Position Dynamics/1(dx1) -> Mux/1
  Demux3/3 -> Rotation Dynamics/3(x3)
  Demux3/5 -> Rotation Dynamics/5(x5)
  Rotation Dynamics/3(dx9) -> Mux2/3
  Demux4/6 -> Rotation Dynamics/12(x12)
  Rotation Dynamics/5(dx11) -> Mux2/5
  Mux5/1 -> "x7, x9, x11"/1, Terminator1/1  "x7, x9, x11"
  Demux4/2 -> Rotation Dynamics/8(x8)
  Mux1/1 -> Integrator/1  "dx"
  Rotation Dynamics/2(dx8) -> Sum/2
  Sum/1 -> Mux2/2
  Mux3/1 -> To Workspace/1, Scope/1
  Mux4/1 -> Scope1/1, To Workspace1/1
  Rotation Dynamics/4(dx10) -> Sum1/2
  Sum1/1 -> Mux2/4
  Sum2/1 -> Mux2/6
  Rotation Dynamics/6(dx12) -> Sum2/2
  Angle Disturbances/1 -> Demux6/1
  Demux6/1 -> Sum/1  "roll disturbance"
  Demux6/2 -> Sum1/1  "pitch disturbance"
  Demux6/3 -> Sum2/1  "yaw disturbance"
  Position Dynamics/2(dx2) -> Sum3/2
  Sum3/1 -> Mux/2
  Position Dynamics/4(dx4) -> Sum4/2
  Sum4/1 -> Mux/4
  Sum5/1 -> Mux/6
  Position Dynamics/6(dx6) -> Sum5/2
  Mux6/1 -> Drag and Wind Disturbances/2(vi)  "vi"
  Mux7/1 -> Drag and Wind Disturbances/3(Input1)
  Drag and Wind Disturbances/1(Out1) -> Sum3/1
  Drag and Wind Disturbances/2(Out2) -> Sum4/1
  Drag and Wind Disturbances/3(Out3) -> Sum5/1
  Wind Disturbances/1 -> Drag and Wind Disturbances/1(Input)

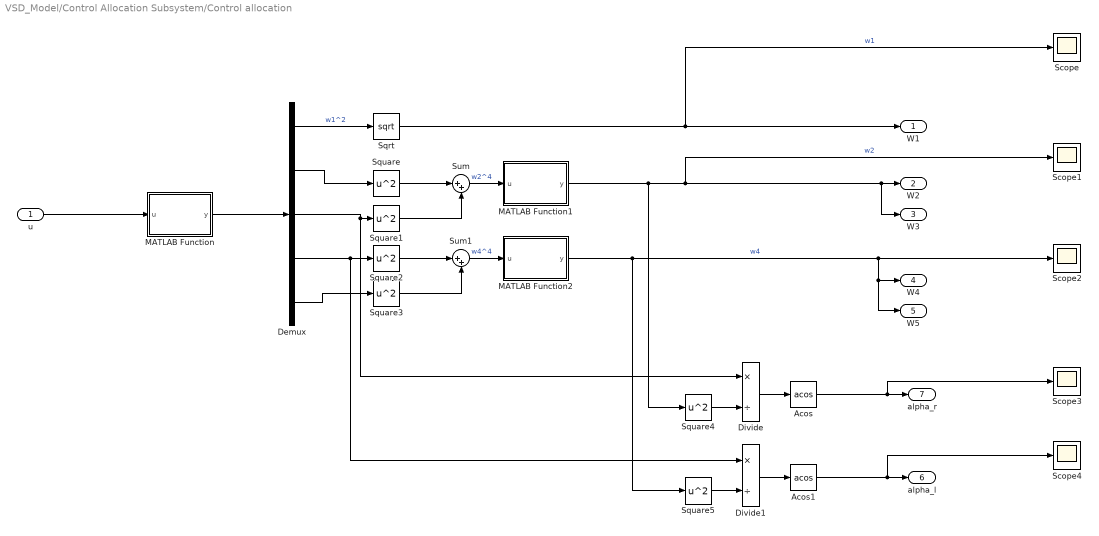
== system VSD_Model/Control Allocation Subsystem/Control allocation ==
  u : Inport
  Acos : Trigonometry  Operator=acos
  Acos1 : Trigonometry  Operator=acos
  Demux : Demux  Outputs=5
  Divide : Product  Inputs=*/
  Divide1 : Product  Inputs=*/
  MATLAB Function : MATLAB Function  TreatAsAtomicUnit=on
  MATLAB Function1 : MATLAB Function  TreatAsAtomicUnit=on
  MATLAB Function2 : MATLAB Function  TreatAsAtomicUnit=on
  Scope{,1..4} (5 alike) : Scope
  Sqrt : Sqrt
  Square{,1..5} (6 alike) : Math  Operator=square
  Sum : Sum  Inputs=|++
  Sum1 : Sum  Inputs=|++
  W1 : Outport
  W2 : Outport  Port=2
  W3 : Outport  Port=3
  W4 : Outport  Port=4
  W5 : Outport  Port=5
  alpha_l : Outport  Port=6
  alpha_r : Outport  Port=7
  wires:
  u/1 -> MATLAB Function/1(u)
  MATLAB Function/1(y) -> Demux/1
  Demux/1 -> Sqrt/1  "w1^2"
  Sqrt/1 -> W1/1, Scope/1  "w1"
  Demux/2 -> Square/1
  Demux/3 -> Divide/1, Square1/1
  Square/1 -> Sum/1
  Square1/1 -> Sum/2
  Sum/1 -> MATLAB Function1/1(u)  "w2^4"
  MATLAB Function1/1(y) -> Square4/1, W3/1, W2/1, Scope1/1  "w2"
  Square3/1 -> Sum1/2
  Demux/5 -> Square3/1
  Demux/4 -> Divide1/1, Square2/1
  Square2/1 -> Sum1/1
  Sum1/1 -> MATLAB Function2/1(u)  "w4^4"
  MATLAB Function2/1(y) -> W5/1, W4/1, Scope2/1, Square5/1  "w4"
  Square4/1 -> Divide/2
  Divide/1 -> Acos/1
  Acos/1 -> Scope3/1, alpha_r/1
  Square5/1 -> Divide1/2
  Divide1/1 -> Acos1/1
  Acos1/1 -> Scope4/1, alpha_l/1

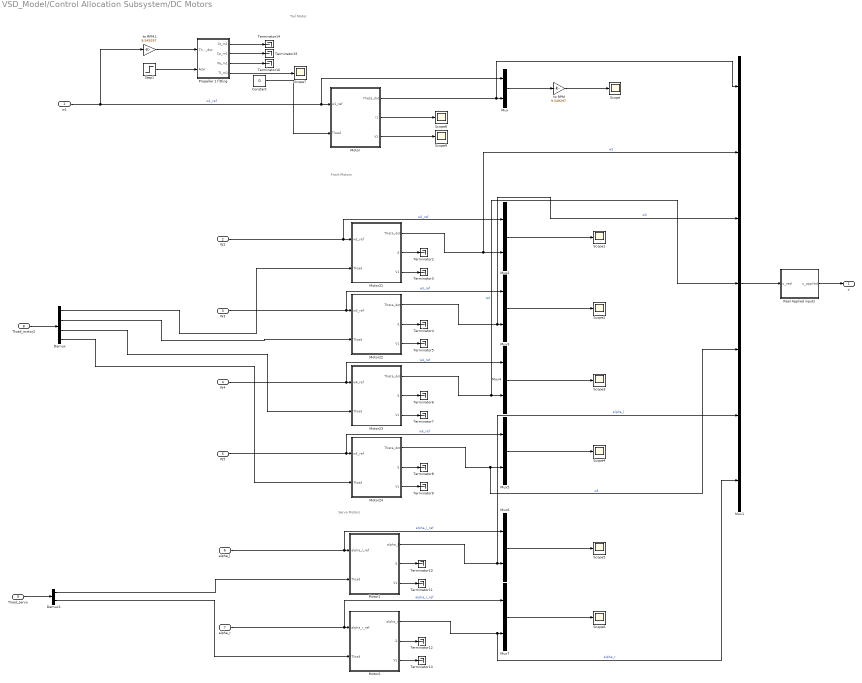
== system VSD_Model/Control Allocation Subsystem/DC Motors ==
  note: Front Motors
  note: Servo Motors
  note: Tail Motor
  w1 : Inport
  W2 : Inport  Port=2
  W3 : Inport  Port=3
  W4 : Inport  Port=4
  W5 : Inport  Port=5
  alpha_l : Inport  Port=6
  alpha_r : Inport  Port=7
  Tload_motor2 : Inport  Port=8
  Tload_servo : Inport  Port=9
  Constant : Constant  Value=0
  Demux : Demux
  Demux1 : Demux  Outputs=2
  Motor : Subsystem
  Motor1 : Subsystem
  Motor2 : Subsystem
  Motor21 : Subsystem
  Motor22 : Subsystem
  Motor23 : Subsystem
  Motor24 : Subsystem
  Mux{,2..7} (7 alike) : Mux  Inputs=2
  Mux1 : Mux  Inputs=7
  Propeller 1 fitting : Subsystem
  Real Applied inputs : MATLAB Function  TreatAsAtomicUnit=on
  Scope{,1..9} (10 alike) : Scope
  Step1 : Step  Time=0  After=0.5  SampleTime=0
  Terminator{2..16} (15 alike) : Terminator
  to RPM : Gain  Gain=9.549297
  to RPM1 : Gain  Gain=9.549297
  y : Outport
  wires:
  Mux2/1 -> Scope1/1
  Mux3/1 -> Scope2/1
  Mux4/1 -> Scope3/1
  Mux5/1 -> Scope4/1
  Mux1/1 -> Real Applied inputs/1(u_real)
  Real Applied inputs/1(u_applied) -> y/1
  alpha_l/1 -> Mux6/1, Motor1/1(alpha_l_ref)  "alpha_l_ref"
  Mux6/1 -> Scope5/1
  alpha_r/1 -> Mux7/1, Motor2/1(alpha_r_ref)  "alpha_r_ref"
  Mux7/1 -> Scope6/1
  w1/1 -> to RPM1/1, Motor/1(w1_ref), Mux/1  "w1_ref"
  Motor/1(Theta_dot) -> Mux1/1, Mux/2
  Motor/3(V1) -> Scope9/1
  Tload_motor2/1 -> Demux/1
  W2/1 -> Motor21/1(w1_ref), Mux2/1  "w2_ref"
  Motor21/1(Theta_dot) -> Mux2/2, Mux1/2  "w2"
  Motor21/2(i1) -> Terminator2/1
  Motor21/3(V1) -> Terminator3/1
  Motor22/3(V1) -> Terminator5/1
  Motor22/2(i1) -> Terminator4/1
  Motor22/1(Theta_dot) -> Mux1/3, Mux3/2  "w3"
  W3/1 -> Mux3/1, Motor22/1(w3_ref)  "w3_ref"
  Motor23/2(i1) -> Terminator6/1
  Motor23/3(V1) -> Terminator7/1
  Motor23/1(Theta_dot) -> Mux1/4, Mux4/2  "w4"
  W4/1 -> Mux4/1, Motor23/1(w4_ref)  "w4_ref"
  Motor24/2(i1) -> Terminator8/1
  Motor24/3(V1) -> Terminator9/1
  W5/1 -> Motor24/1(w5_ref), Mux5/1  "w5_ref"
  Motor24/1(Theta_dot) -> Mux1/5, Mux5/2  "w5"
  Motor1/2(i1) -> Terminator10/1
  Motor1/3(V1) -> Terminator11/1
  Motor1/1(alpha_l) -> Mux1/6, Mux6/2  "alpha_l"
  Motor2/3(V1) -> Terminator13/1
  Motor2/2(i1) -> Terminator12/1
  Motor2/1(alpha_r) -> Mux1/7, Mux7/2  "alpha_r"
  Demux/1 -> Motor21/2(Tload)
  Demux/2 -> Motor22/2(Tload)
  Demux/3 -> Motor23/2(Tload)
  Demux/4 -> Motor24/2(Tload)
  Tload_servo/1 -> Demux1/1
  Demux1/1 -> Motor1/2(Tload)
  Demux1/2 -> Motor2/2(Tload)
  to RPM/1 -> Scope/1
  Mux/1 -> to RPM/1
  Step1/1 -> Propeller 1 fitting/2(Advr)
  Propeller 1 fitting/1(Ct_m1) -> Terminator14/1
  Propeller 1 fitting/4(Tl_m1) -> Scope7/1
  Propeller 1 fitting/3(Pe_m1) -> Terminator16/1
  Propeller 1 fitting/2(Cp_m1) -> Terminator15/1
  to RPM1/1 -> Propeller 1 fitting/1(Theta_dot)
  Motor/2(i1) -> Scope8/1
  Constant/1 -> Motor/2(Tload)

== system VSD_Model/Reference Generator/Pitch Yaw Reference Generator ==
  Mux : Mux  Inputs=2
  To Workspace : ToWorkspace  VariableName=x9r  SampleTime=-1
  To Workspace1 : ToWorkspace  VariableName=x11r  SampleTime=-1
  x11r1 : Step  Time=0  After=0  SampleTime=0
  x9r : Step  Time=0  After=0.5  SampleTime=0
  "x9r, x11r" : Outport
  wires:
  x9r/1 -> To Workspace/1, Mux/1  "desired pitch angle"
  x11r1/1 -> To Workspace1/1, Mux/2  "desired yaw angle"
  Mux/1 -> "x9r, x11r"/1

== system VSD_Model/Sensors Model1/Subsystem ==
  y : Inport
  x : Inport  Port=2
  Demux : Demux  Outputs=12
  Demux1 : Demux  Outputs=12
  Mux : Mux  Inputs=2
  Mux1 : Mux  Inputs=2
  Mux2 : Mux  Inputs=2
  Scope : Scope
  Scope1 : Scope
  Scope2 : Scope
  wires:
  y/1 -> Demux/1
  x/1 -> Demux1/1
  Mux/1 -> Scope/1
  Demux/1 -> Mux/1
  Demux1/1 -> Mux/2
  Mux1/1 -> Scope1/1
  Demux/7 -> Mux1/1
  Demux1/7 -> Mux1/2
  Mux2/1 -> Scope2/1
  Demux/8 -> Mux2/1
  Demux1/8 -> Mux2/2

== system VSD_Model/Subsystem/Scopes1 ==
  x : Inport
  y : Inport  Port=2
  xhat_EKF : Inport  Port=3
  xhat_UKF : Inport  Port=4
  Demux : Demux  Outputs=12
  Demux1 : Demux  Outputs=12
  Demux2 : Demux  Outputs=6
  Demux3 : Demux  Outputs=12
  Mux : Mux
  Scope : Scope
  wires:
  x/1 -> Demux/1
  xhat_EKF/1 -> Demux1/1
  Demux/2 -> Mux/1
  Demux1/2 -> Mux/2  "xhat_EKF"
  Mux/1 -> Scope/1
  y/1 -> Demux2/1
  xhat_UKF/1 -> Demux3/1
  Demux3/2 -> Mux/3  "xhat_UKF"
  Demux2/1 -> Mux/4  "y"

== system VSD_Model/Subsystem/Sensors Model2 ==
  x_if : Inport
  Body 2 Inertial : MATLAB Function  TreatAsAtomicUnit=on
  Demux : Demux  Outputs=12
  Demux1 : Demux  Outputs=3
  Demux2 : Demux  Outputs=3
  From Body to Inertial Coordinates : MATLAB Function  TreatAsAtomicUnit=on
  From Inertial to Body Coordinates : MATLAB Function  TreatAsAtomicUnit=on
  Measurments Noise (Angular Rates) : simulink/Sources/Band-Limited White Noise  Cov=R*Ts  Ts=Ts  seed=[23341]
  Measurments Noise (Angular Rates)1 : simulink/Sources/Band-Limited White Noise  Cov=R*Ts  Ts=Ts  seed=[23341]
  Mux : Mux  Inputs=12
  Mux1 : Mux  Inputs=6
  Sum : Sum  Inputs=++|
  Sum1 : Sum  Inputs=++|
  y_withNoise : Outport
  wires:
  x_if/1 -> From Inertial to Body Coordinates/1(x_if), From Body to Inertial Coordinates/2(x_if), Body 2 Inertial/2(x_if), Demux/1
  From Inertial to Body Coordinates/2(omega_bf) -> Sum/2
  From Inertial to Body Coordinates/1(v_bf) -> Sum1/2
  Measurments Noise (Angular Rates)1/1 -> Sum1/1
  Measurments Noise (Angular Rates)/1 -> Sum/1
  Sum1/1 -> From Body to Inertial Coordinates/1(u)  "translational speeds with Noise"
  Sum/1 -> Body 2 Inertial/1(u)  "angular rates with Noise"
  From Body to Inertial Coordinates/1(y) -> Demux1/1
  Body 2 Inertial/1(y) -> Demux2/1
  Demux2/3 -> Mux1/6, Mux/12
  Demux2/2 -> Mux/10, Mux1/5
  Demux2/1 -> Mux/8, Mux1/4
  Demux/11 -> Mux/11
  Demux/9 -> Mux/9
  Demux/7 -> Mux/7
  Demux/1 -> Mux/1
  Demux/3 -> Mux/3
  Demux/5 -> Mux/5
  Demux1/1 -> Mux1/1, Mux/2
  Demux1/2 -> Mux/4, Mux1/2
  Demux1/3 -> Mux/6, Mux1/3
  Mux1/1 -> y_withNoise/1

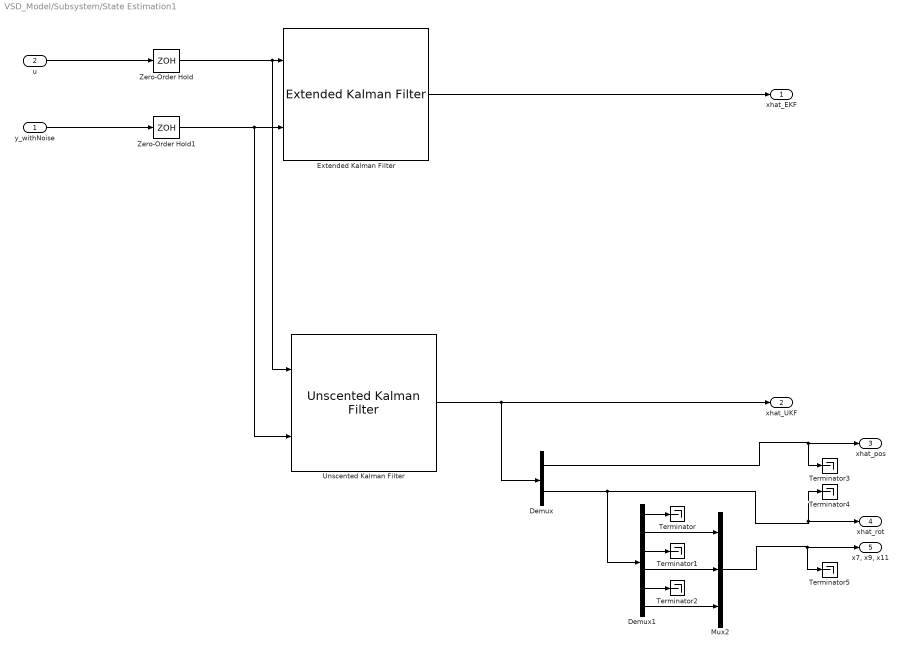
== system VSD_Model/Subsystem/State Estimation1 ==
  y_withNoise : Inport
  u : Inport  Port=2
  Demux : Demux  Outputs=2
  Demux1 : Demux  Outputs=6
  Extended Kalman Filter : sharedTrackingLibrary/Extended Kalman Filter  StateTransitionFcn=myStateTransitionFcn  HasStateTransitionJacobianFcn=off  HasAdditiveProcessNoise=Additive  ProcessNoise=Q*eye(12)  HasTimeVaryingProcessNoise=off  HasStateTransitionFcnExtraArgument=1  InitialState=x0  InitialStateCovariance=1e-6  MeasurementFcn1=myMeasurementFcn  HasMeasurementJacobianFcn1=off  HasMeasurementEnablePort1=off  HasAdditiveMeasurementNoise1=Additive  MeasurementNoise1=R*eye(6)  HasTimeVaryingMeasurementNoise1=off  HasMeasurementFcnExtraArgument1=0  HasMeasurementWrapping1=off  MeasurementFcn2=myMeasurementFcn  HasMeasurementJacobianFcn2=off  HasMeasurementEnablePort2=off  HasAdditiveMeasurementNoise2=Additive  MeasurementNoise2=1  HasTimeVaryingMeasurementNoise2=off  HasMeasurementFcnExtraArgument2=0  HasMeasurementWrapping2=off  MeasurementFcn3=myMeasurementFcn  HasMeasurementJacobianFcn3=off  HasMeasurementEnablePort3=off  HasAdditiveMeasurementNoise3=Additive  MeasurementNoise3=1  HasTimeVaryingMeasurementNoise3=off  HasMeasurementFcnExtraArgument3=0  HasMeasurementWrapping3=off  MeasurementFcn4=myMeasurementFcn  HasMeasurementJacobianFcn4=off  HasMeasurementEnablePort4=off  HasAdditiveMeasurementNoise4=Additive  MeasurementNoise4=1  HasTimeVaryingMeasurementNoise4=off  HasMeasurementFcnExtraArgument4=0  HasMeasurementWrapping4=off  MeasurementFcn5=myMeasurementFcn  HasMeasurementJacobianFcn5=off  HasMeasurementEnablePort5=off  HasAdditiveMeasurementNoise5=Additive  MeasurementNoise5=1  HasTimeVaryingMeasurementNoise5=off  HasMeasurementFcnExtraArgument5=0  HasMeasurementWrapping5=off  EnableMultirate=off  StateTransitionFcnSampleTime=1  MeasurementFcn1SampleTime=1  MeasurementFcn2SampleTime=1  MeasurementFcn3SampleTime=1  MeasurementFcn4SampleTime=1  MeasurementFcn5SampleTime=1  UseCurrentEstimator=on  OutputStateCovariance=off  DataType=double  SampleTime=Ts  NumberOfMeasurements=1
      settings: SourceProductBaseCode=TF,AE,PW,CT,DR,ID,LP,NV,AR,RO,RR,UV,VE
  Mux2 : Mux  Inputs=3
  Terminator{,1..5} (6 alike) : Terminator
  Unscented Kalman Filter : sharedTrackingLibrary/Unscented Kalman Filter  StateTransitionFcn=myStateTransitionFcn  HasAdditiveProcessNoise=Additive  ProcessNoise=Q*eye(12)  HasTimeVaryingProcessNoise=off  HasStateTransitionFcnExtraArgument=1  InitialState=x0  InitialStateCovariance=1e-6  Alpha=1e-3  Beta=2  Kappa=0  MeasurementFcn1=myMeasurementFcn  HasMeasurementEnablePort1=off  HasAdditiveMeasurementNoise1=Additive  MeasurementNoise1=R*eye(6)  HasTimeVaryingMeasurementNoise1=off  HasMeasurementFcnExtraArgument1=0  HasMeasurementWrapping1=off  MeasurementFcn2=myMeasurementFcn  HasMeasurementEnablePort2=off  HasAdditiveMeasurementNoise2=Additive  MeasurementNoise2=1  HasTimeVaryingMeasurementNoise2=off  HasMeasurementFcnExtraArgument2=0  HasMeasurementWrapping2=off  MeasurementFcn3=myMeasurementFcn  HasMeasurementEnablePort3=off  HasAdditiveMeasurementNoise3=Additive  MeasurementNoise3=1  HasTimeVaryingMeasurementNoise3=off  HasMeasurementFcnExtraArgument3=0  HasMeasurementWrapping3=off  MeasurementFcn4=myMeasurementFcn  HasMeasurementEnablePort4=off  HasAdditiveMeasurementNoise4=Additive  MeasurementNoise4=1  HasTimeVaryingMeasurementNoise4=off  HasMeasurementFcnExtraArgument4=0  HasMeasurementWrapping4=off  MeasurementFcn5=myMeasurementFcn  HasMeasurementEnablePort5=off  HasAdditiveMeasurementNoise5=Additive  MeasurementNoise5=1  HasTimeVaryingMeasurementNoise5=off  HasMeasurementFcnExtraArgument5=0  HasMeasurementWrapping5=off  EnableMultirate=off  StateTransitionFcnSampleTime=1  MeasurementFcn1SampleTime=1  MeasurementFcn2SampleTime=1  MeasurementFcn3SampleTime=1  MeasurementFcn4SampleTime=1  MeasurementFcn5SampleTime=1  UseCurrentEstimator=on  OutputStateCovariance=off  DataType=double  SampleTime=Ts  NumberOfMeasurements=1
      settings: SourceProductBaseCode=TF,AE,PW,CT,DR,ID,LP,NV,AR,RO,RR,UV,VE
  Zero-Order Hold : ZeroOrderHold  SampleTime=Ts
  Zero-Order Hold1 : ZeroOrderHold  SampleTime=Ts
  xhat_EKF : Outport
  xhat_UKF : Outport  Port=2
  xhat_pos : Outport  Port=3
  xhat_rot : Outport  Port=4
  "x7, x9, x11" : Outport  Port=5
  wires:
  u/1 -> Zero-Order Hold/1
  Zero-Order Hold/1 -> Unscented Kalman Filter/1, Extended Kalman Filter/1
  y_withNoise/1 -> Zero-Order Hold1/1
  Zero-Order Hold1/1 -> Unscented Kalman Filter/2, Extended Kalman Filter/2
  Extended Kalman Filter/1 -> xhat_EKF/1
  Demux/1 -> Terminator3/1, xhat_pos/1
  Demux/2 -> Terminator4/1, xhat_rot/1, Demux1/1
  Demux1/1 -> Terminator/1
  Demux1/3 -> Terminator1/1
  Demux1/5 -> Terminator2/1
  Demux1/2 -> Mux2/1
  Demux1/4 -> Mux2/2
  Demux1/6 -> Mux2/3
  Mux2/1 -> Terminator5/1, "x7, x9, x11"/1
  Unscented Kalman Filter/1 -> xhat_UKF/1, Demux/1

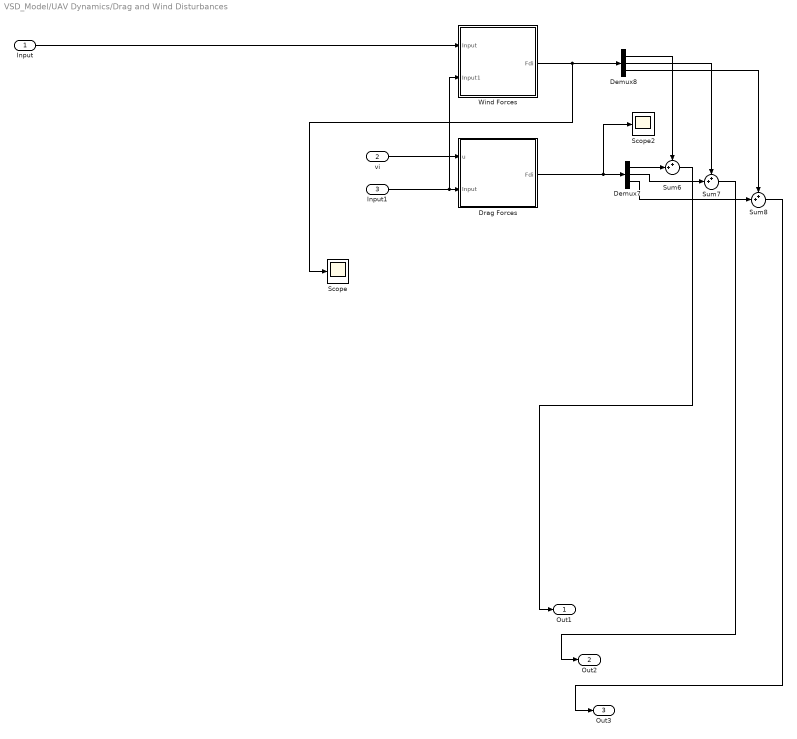
== system VSD_Model/UAV Dynamics/Drag and Wind Disturbances ==
  Input : Inport
  vi : Inport  Port=2
  Input1 : Inport  Port=3
  Demux7 : Demux  Outputs=3
  Demux8 : Demux  Outputs=3
  Drag Forces : Subsystem
  Scope : Scope
  Scope2 : Scope
  Sum6 : Sum  Inputs=++|
  Sum7 : Sum  Inputs=++|
  Sum8 : Sum  Inputs=++|
  Wind Forces : Subsystem
  Out1 : Outport
  Out2 : Outport  Port=2
  Out3 : Outport  Port=3
  wires:
  Drag Forces/1(Fdi) -> Scope2/1, Demux7/1
  Input1/1 -> Wind Forces/2(Input1), Drag Forces/2(Input)
  Wind Forces/1(Fdi) -> Scope/1, Demux8/1
  Demux8/2 -> Sum7/1
  Demux8/1 -> Sum6/1
  Demux7/1 -> Sum6/2
  Demux7/2 -> Sum7/2
  Demux8/3 -> Sum8/1
  Demux7/3 -> Sum8/2
  vi/1 -> Drag Forces/1(u)
  Sum7/1 -> Out2/1
  Sum8/1 -> Out3/1
  Sum6/1 -> Out1/1
  Input/1 -> Wind Forces/1(Input)

== system VSD_Model/Control Allocation Subsystem/DC Motors/Motor ==
  w1_ref : Inport
  Tload : Inport  Port=2
  DC Motor : Subsystem
  PID Controller : slpidlib/PID Controller  Controller=PID  Form=Parallel  TimeDomain=Continuous-time  UseExternalTs=off  SampleTime=-1  IntegratorMethod=Forward Euler  FilterMethod=Forward Euler  ControllerParametersSource=internal  P=0.0221631801492144  I=0.197988325342969  UseKiTs=off  D=-5.9672220338915e-06  N=3714.15375920925  UseFilter=on  TunerSelectOption=Transfer Function Based (PID Tuner App)  InitialConditionSource=internal  InitialConditionForIntegrator=0  InitialConditionForFilter=0  DifferentiatorICPrevScaledInput=0  ExternalReset=none  TrackingMode=off  Kt=1  LimitOutput=off  SatLimitsSource=internal  UpperSaturationLimit=inf  LowerSaturationLimit=-inf  LinearizeAsGain=on  AntiWindupMode=none  Kb=1  POutMin=[]  POutMax=[]  IOutMin=[]  IOutMax=[]  DOutMin=[]  DOutMax=[]  NOutMin=[]  NOutMax=[]  SumOutMin=[]  SumOutMax=[]  SaturationOutMin=[]  SaturationOutMax=[]  PParamMin=[]  PParamMax=[]  IParamMin=[]  IParamMax=[]  DParamMin=[]  DParamMax=[]  NParamMin=[]  NParamMax=[]  KbParamMin=[]  KbParamMax=[]  KtParamMin=[]  KtParamMax=[]  KbOutMin=[]  KbOutMax=[]  KtOutMin=[]  KtOutMax=[]  IntegratorOutMin=[]  IntegratorOutMax=[]  FilterOutMin=[]  FilterOutMax=[]  SumI1OutMin=[]  SumI1OutMax=[]  SumI2OutMin=[]  SumI2OutMax=[]  SumI3OutMin=[]  SumI3OutMax=[]  SumI4OutMin=[]  SumI4OutMax=[]  SumDOutMin=[]  SumDOutMax=[]  DifferentiatorOutMin=[]  DifferentiatorOutMax=[]  FilterDiffOutCoefMin=[]  FilterDiffOutCoefMax=[]  ReciprocalOutMin=[]  ReciprocalOutMax=[]  SumDenOutMin=[]  SumDenOutMax=[]  SumNumOutMin=[]  SumNumOutMax=[]  DivideOutMin=[]  DivideOutMax=[]  UdiffTsProdOutMin=[]  UdiffTsProdOutMax=[]  NTsProdOutMin=[]  NTsProdOutMax=[]  UintegralTsProdOutMin=[]  UintegralTsProdOutMax=[]  UngainTsProdOutMin=[]  UngainTsProdOutMax=[]  IntegratorContinuousStateAttributes=''  IntegratorStateMustResolveToSignalObject=off  IntegratorRTWStateStorageClass=Auto  FilterContinuousStateAttributes=''  FilterStateMustResolveToSignalObject=off  FilterRTWStateStorageClass=Auto  ParallelPVariant=InternalParameters  IdealPVariant=Disabled  IVariant=InternalParameters  DVariant=InternalParameters  IntegratorVariant=Continuous  SatVariant=Disabled  AWVariant=Passthrough  PCopyVariant=Disabled  TRVariant=Disabled  FdbkBlocksVariant=Forward  IdealPFdbkVariant=Disabled  SatFdbkVariant=Disabled  DerivativeFilterVariant=ContFilter  NVariant=InternalParameters  NCopyVariant=Disabled  FilterICVariant=InternalICsFilter  IntegratorICVariant=InternalICs  ExternalResetVariant=Disabled  TRSumVariant=Passthrough  SumFdbkVariant=Disabled  SumVariant=Sum_PID  TsampFilterVariant=InternalTs  TsampNgainVariant=Passthrough  TsampIntegralVariant=Passthrough  ExternalSaturationOutDataTypeStr=Inherit: Same as second input  aMode=0
  Step : Step  Time=0  After=0.0015  SampleTime=0
  Sum : Sum  Inputs=|+-
  Theta_dot : Outport
  i1 : Outport  Port=2
  V1 : Outport  Port=3
  wires:
  Sum/1 -> PID Controller/1
  Tload/1 -> DC Motor/2(Tload)
  Step/1 -> DC Motor/3(T_S)
  PID Controller/1 -> DC Motor/1(Vm), V1/1
  DC Motor/2(ia) -> i1/1
  w1_ref/1 -> Sum/1
  DC Motor/1(Theta_dot) -> Theta_dot/1, Sum/2

== system VSD_Model/Control Allocation Subsystem/DC Motors/Motor1 ==
  alpha_l_ref : Inport
  Tload : Inport  Port=2
  DC Motor : Subsystem
  PID Controller : slpidlib/PID Controller  Controller=PID  Form=Parallel  TimeDomain=Continuous-time  UseExternalTs=off  SampleTime=-1  IntegratorMethod=Forward Euler  FilterMethod=Forward Euler  ControllerParametersSource=internal  P=0.0215432440144619  I=0.00427711815263808  UseKiTs=off  D=0.0241097065819863  N=3889.19643311843  UseFilter=on  TunerSelectOption=Transfer Function Based (PID Tuner App)  InitialConditionSource=internal  InitialConditionForIntegrator=0  InitialConditionForFilter=0  DifferentiatorICPrevScaledInput=0  ExternalReset=none  TrackingMode=off  Kt=1  LimitOutput=off  SatLimitsSource=internal  UpperSaturationLimit=inf  LowerSaturationLimit=-inf  LinearizeAsGain=on  AntiWindupMode=none  Kb=1  POutMin=[]  POutMax=[]  IOutMin=[]  IOutMax=[]  DOutMin=[]  DOutMax=[]  NOutMin=[]  NOutMax=[]  SumOutMin=[]  SumOutMax=[]  SaturationOutMin=[]  SaturationOutMax=[]  PParamMin=[]  PParamMax=[]  IParamMin=[]  IParamMax=[]  DParamMin=[]  DParamMax=[]  NParamMin=[]  NParamMax=[]  KbParamMin=[]  KbParamMax=[]  KtParamMin=[]  KtParamMax=[]  KbOutMin=[]  KbOutMax=[]  KtOutMin=[]  KtOutMax=[]  IntegratorOutMin=[]  IntegratorOutMax=[]  FilterOutMin=[]  FilterOutMax=[]  SumI1OutMin=[]  SumI1OutMax=[]  SumI2OutMin=[]  SumI2OutMax=[]  SumI3OutMin=[]  SumI3OutMax=[]  SumI4OutMin=[]  SumI4OutMax=[]  SumDOutMin=[]  SumDOutMax=[]  DifferentiatorOutMin=[]  DifferentiatorOutMax=[]  FilterDiffOutCoefMin=[]  FilterDiffOutCoefMax=[]  ReciprocalOutMin=[]  ReciprocalOutMax=[]  SumDenOutMin=[]  SumDenOutMax=[]  SumNumOutMin=[]  SumNumOutMax=[]  DivideOutMin=[]  DivideOutMax=[]  UdiffTsProdOutMin=[]  UdiffTsProdOutMax=[]  NTsProdOutMin=[]  NTsProdOutMax=[]  UintegralTsProdOutMin=[]  UintegralTsProdOutMax=[]  UngainTsProdOutMin=[]  UngainTsProdOutMax=[]  IntegratorContinuousStateAttributes=''  IntegratorStateMustResolveToSignalObject=off  IntegratorRTWStateStorageClass=Auto  FilterContinuousStateAttributes=''  FilterStateMustResolveToSignalObject=off  FilterRTWStateStorageClass=Auto  ParallelPVariant=InternalParameters  IdealPVariant=Disabled  IVariant=InternalParameters  DVariant=InternalParameters  IntegratorVariant=Continuous  SatVariant=Disabled  AWVariant=Passthrough  PCopyVariant=Disabled  TRVariant=Disabled  FdbkBlocksVariant=Forward  IdealPFdbkVariant=Disabled  SatFdbkVariant=Disabled  DerivativeFilterVariant=ContFilter  NVariant=InternalParameters  NCopyVariant=Disabled  FilterICVariant=InternalICsFilter  IntegratorICVariant=InternalICs  ExternalResetVariant=Disabled  TRSumVariant=Passthrough  SumFdbkVariant=Disabled  SumVariant=Sum_PID  TsampFilterVariant=InternalTs  TsampNgainVariant=Passthrough  TsampIntegralVariant=Passthrough  ExternalSaturationOutDataTypeStr=Inherit: Same as second input  aMode=0
  Step : Step  Time=0  After=0.0015  SampleTime=0
  Sum : Sum  Inputs=|+-
  alpha_l : Outport
  i1 : Outport  Port=2
  V1 : Outport  Port=3
  wires:
  Sum/1 -> PID Controller/1
  Tload/1 -> DC Motor/2(Tload)
  Step/1 -> DC Motor/3(T_S)
  PID Controller/1 -> DC Motor/1(Vm), V1/1
  DC Motor/2(ia) -> i1/1
  alpha_l_ref/1 -> Sum/1
  DC Motor/1(alpha_l) -> alpha_l/1, Sum/2

== system VSD_Model/Control Allocation Subsystem/DC Motors/Motor2 ==
  alpha_r_ref : Inport
  Tload : Inport  Port=2
  DC Motor : Subsystem
  PID Controller : slpidlib/PID Controller  Controller=PID  Form=Parallel  TimeDomain=Continuous-time  UseExternalTs=off  SampleTime=-1  IntegratorMethod=Forward Euler  FilterMethod=Forward Euler  ControllerParametersSource=internal  P=0.191362495500226  I=0.35975303585234  UseKiTs=off  D=0.0236909641348743  N=72.2455805470514  UseFilter=on  TunerSelectOption=Transfer Function Based (PID Tuner App)  InitialConditionSource=internal  InitialConditionForIntegrator=0  InitialConditionForFilter=0  DifferentiatorICPrevScaledInput=0  ExternalReset=none  TrackingMode=off  Kt=1  LimitOutput=off  SatLimitsSource=internal  UpperSaturationLimit=inf  LowerSaturationLimit=-inf  LinearizeAsGain=on  AntiWindupMode=none  Kb=1  POutMin=[]  POutMax=[]  IOutMin=[]  IOutMax=[]  DOutMin=[]  DOutMax=[]  NOutMin=[]  NOutMax=[]  SumOutMin=[]  SumOutMax=[]  SaturationOutMin=[]  SaturationOutMax=[]  PParamMin=[]  PParamMax=[]  IParamMin=[]  IParamMax=[]  DParamMin=[]  DParamMax=[]  NParamMin=[]  NParamMax=[]  KbParamMin=[]  KbParamMax=[]  KtParamMin=[]  KtParamMax=[]  KbOutMin=[]  KbOutMax=[]  KtOutMin=[]  KtOutMax=[]  IntegratorOutMin=[]  IntegratorOutMax=[]  FilterOutMin=[]  FilterOutMax=[]  SumI1OutMin=[]  SumI1OutMax=[]  SumI2OutMin=[]  SumI2OutMax=[]  SumI3OutMin=[]  SumI3OutMax=[]  SumI4OutMin=[]  SumI4OutMax=[]  SumDOutMin=[]  SumDOutMax=[]  DifferentiatorOutMin=[]  DifferentiatorOutMax=[]  FilterDiffOutCoefMin=[]  FilterDiffOutCoefMax=[]  ReciprocalOutMin=[]  ReciprocalOutMax=[]  SumDenOutMin=[]  SumDenOutMax=[]  SumNumOutMin=[]  SumNumOutMax=[]  DivideOutMin=[]  DivideOutMax=[]  UdiffTsProdOutMin=[]  UdiffTsProdOutMax=[]  NTsProdOutMin=[]  NTsProdOutMax=[]  UintegralTsProdOutMin=[]  UintegralTsProdOutMax=[]  UngainTsProdOutMin=[]  UngainTsProdOutMax=[]  IntegratorContinuousStateAttributes=''  IntegratorStateMustResolveToSignalObject=off  IntegratorRTWStateStorageClass=Auto  FilterContinuousStateAttributes=''  FilterStateMustResolveToSignalObject=off  FilterRTWStateStorageClass=Auto  ParallelPVariant=InternalParameters  IdealPVariant=Disabled  IVariant=InternalParameters  DVariant=InternalParameters  IntegratorVariant=Continuous  SatVariant=Disabled  AWVariant=Passthrough  PCopyVariant=Disabled  TRVariant=Disabled  FdbkBlocksVariant=Forward  IdealPFdbkVariant=Disabled  SatFdbkVariant=Disabled  DerivativeFilterVariant=ContFilter  NVariant=InternalParameters  NCopyVariant=Disabled  FilterICVariant=InternalICsFilter  IntegratorICVariant=InternalICs  ExternalResetVariant=Disabled  TRSumVariant=Passthrough  SumFdbkVariant=Disabled  SumVariant=Sum_PID  TsampFilterVariant=InternalTs  TsampNgainVariant=Passthrough  TsampIntegralVariant=Passthrough  ExternalSaturationOutDataTypeStr=Inherit: Same as second input  aMode=0
  Step : Step  Time=0  After=0.0015  SampleTime=0
  Sum : Sum  Inputs=|+-
  alpha_r : Outport
  i1 : Outport  Port=2
  V1 : Outport  Port=3
  wires:
  Sum/1 -> PID Controller/1
  Tload/1 -> DC Motor/2(Tload)
  Step/1 -> DC Motor/3(T_S)
  PID Controller/1 -> DC Motor/1(Vm), V1/1
  DC Motor/2(ia) -> i1/1
  alpha_r_ref/1 -> Sum/1
  DC Motor/1(Theta) -> alpha_r/1, Sum/2
